simulink model "AC_PotMed"  (R2020a)
settings: Solver=VariableStepAuto  StartTime=0.0  StopTime=1600  MaxStep=0.001  RelTol=1e-3  EnableMultiTasking=on
InitFcn:
  | R=4
  | C=3.6
  | Rm=1
  | Cm=4.3
  | eta=3
  | Tmin=19.5
  | Tmax=20.5
  | P=0.6
  | deltaT=2
libraries: simulink x1
settings Model: Creator=daniel  LastModifiedBy=User
settings SolverCC: ZeroCrossControl=DisableAll
settings DataIOCC: LimitDataPoints=on  ReturnWorkspaceOutputs=off
settings OptimizationCC: LifeSpan=inf
settings DebuggingCC: AllowSymbolicDim=off  SFUnexpectedBacktrackingDiag=warning  SFNoUnconditionalDefaultTransitionDiag=warning  SFExecutionAtInitializationDiag=none  ArithmeticOperatorsInVariantConditions=warning
settings ModelReferenceCC: PropagateSignalLabelsOutOfModel=off
settings SFSimCC: SimUseLocalCustomCode=off  CustomCodeUndefinedFunction=UseInterfaceOnly
settings RTWCC: RTWUseLocalCustomCode=off
settings CodeAppCC: StateflowObjectComments=on
settings GRTTargetCC: TargetLangStandard=C89/C90 (ANSI)
settings ConfigComp: CovMetricSettings=dw  CovHtmlReporting=on  CovSaveCumulativeToWorkspaceVar=on  CovSaveSingleToWorkspaceVar=on  CovExternalEMLEnable=off

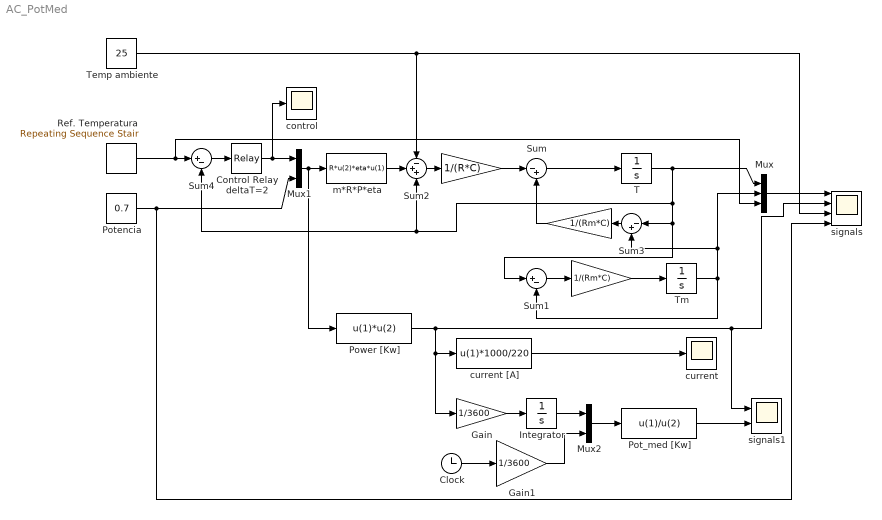
== system AC_PotMed ==
  " " : Gain  Gain=1/(Rm*C)
  "  " : Gain  Gain=1/(Rm*C)
  "   " : Gain  Gain=1/(R*C)
  Clock : Clock
  Control Relay deltaT=2 : Relay  OnSwitchValue=0.5  OffSwitchValue=-0.5  OnOutputValue=0  OffOutputValue=1
  Gain : Gain  Gain=1/3600
  Gain1 : Gain  Gain=1/3600
  Integrator : Integrator
  Mux : Mux  Inputs=3
  Mux1 : Mux  Inputs=2
  Mux2 : Mux  Inputs=2
  Pot_med [Kw] : Fcn  Expr=u(1)/u(2)
  Potencia : Constant  Value=0.7
  Power [Kw] : Fcn  Expr=u(1)*u(2)
  Ref. Temperatura : simulink/Sources/Repeating Sequence Stair  OutValues=[25 24 23 22 21 20 19 18 18].'  tsamp=200  OutMin=[]  OutMax=[]  OutDataTypeStr=double  OutputDataTypeScalingMode=double  OutDataType=fixdt(0,8)  ConRadixGroup=Best Precision: Vector-wise  OutScaling=2^-12
  Sum : Sum  Inputs=|-+
  Sum1 : Sum  Inputs=|+-
  Sum2 : Sum  Inputs=-++
  Sum3 : Sum  Inputs=|-+
  Sum4 : Sum  Inputs=|+-
  T : Integrator  InitialCondition=30
  Temp ambiente : Constant  Value=25
  Tm : Integrator  InitialCondition=30
  control : Scope
  "current " : Scope
  current [A] : Fcn  Expr=u(1)*1000/220
  m*R*P*eta : Fcn  Expr=R*u(2)*eta*u(1)
  signals : Scope  NumInputPorts=4
  signals1 : Scope  NumInputPorts=2
  wires:
  T/1 -> Sum1/1, Sum3/1, Sum4/2, Sum2/3, Mux/1
  Sum/1 -> T/1
  "  "/1 -> Sum/2
  Sum1/1 -> " "/1
  " "/1 -> Tm/1
  Tm/1 -> Mux/2, Sum3/2, Sum1/2
  "   "/1 -> Sum/1
  Sum2/1 -> "   "/1
  Sum3/1 -> "  "/1
  m*R*P*eta/1 -> Sum2/2
  Mux/1 -> signals/1
  Sum4/1 -> Control Relay deltaT=2/1
  Ref. Temperatura/1 -> Mux/3, Sum4/1
  Temp ambiente/1 -> Sum2/1, signals/3
  Potencia/1 -> Mux1/2, signals/4
  Mux1/1 -> m*R*P*eta/1, Power [Kw]/1
  Control Relay deltaT=2/1 -> control/1, Mux1/1
  current [A]/1 -> "current "/1
  Power [Kw]/1 -> Gain/1, current [A]/1, signals1/1, signals/2
  Gain/1 -> Integrator/1
  Mux2/1 -> Pot_med [Kw]/1
  Clock/1 -> Gain1/1
  Gain1/1 -> Mux2/2
  Integrator/1 -> Mux2/1
  Pot_med [Kw]/1 -> signals1/2
